simulink model "BPPID"  (R2021a)
settings: Solver=ode3  StartTime=0  StopTime=2000  FixedStep=0.05  RelTol=1e-3
settings Model: Creator=kunzhong  LastModifiedBy=sx
settings SolverCC: AlgebraicLoopSolver=TrustRegion
settings DataIOCC: SaveFormat=StructureWithTime  ReturnWorkspaceOutputs=off
settings OptimizationCC: LifeSpan=inf
settings DebuggingCC: SFExecutionAtInitializationDiag=none  SFMachineParentedDataDiag=warning  ArithmeticOperatorsInVariantConditions=warning
settings HardwareCC: ProdBitPerSizeT=32  ProdBitPerPtrDiffT=32  ProdWordSize=32  ProdHWDeviceType=Specified
settings SFSimCC: SimUseLocalCustomCode=off  CustomCodeUndefinedFunction=UseInterfaceOnly
settings RTWCC: RTWUseLocalCustomCode=off
settings CodeAppCC: StateflowObjectComments=on
settings SimscapeCC: SimscapeNormalizeSystem=off

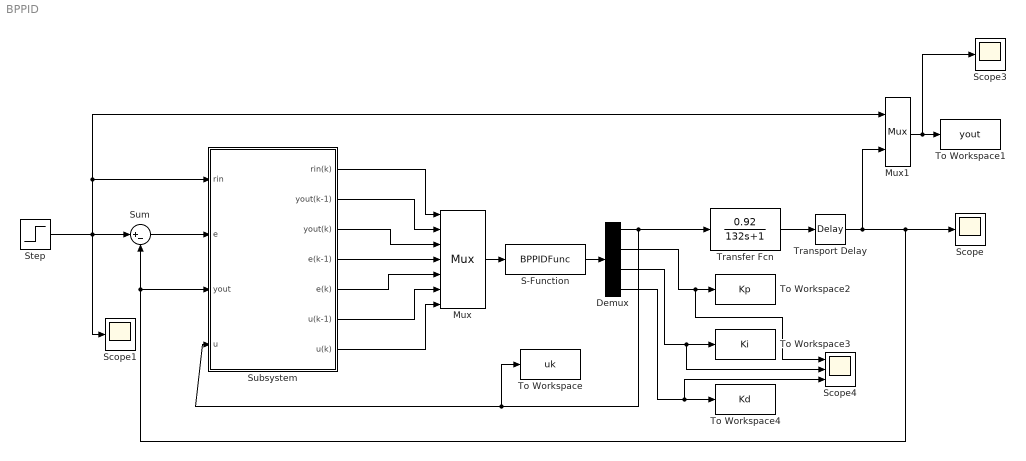
== system BPPID ==
  Demux : Demux
  Mux : Mux  Inputs=7
  Mux1 : Mux  Inputs=2
  S-Function : S-Function  FunctionName=BPPIDFunc  SFunctionDeploymentMode=off  EnableBusSupport=off
  Scope : Scope
  Scope1 : Scope
  Scope3 : Scope
  Scope4 : Scope  NumInputPorts=3
  Step : Step  SampleTime=0  ZeroCross=off
  Subsystem : Subsystem
  Sum : Sum  Inputs=|+-
  To Workspace : ToWorkspace  VariableName=uk  SaveFormat=Structure With Time  SampleTime=-1
  To Workspace1 : ToWorkspace  VariableName=yout  SaveFormat=Structure With Time  SampleTime=-1
  To Workspace2 : ToWorkspace  VariableName=Kp  SaveFormat=Structure With Time  SampleTime=-1
  To Workspace3 : ToWorkspace  VariableName=Ki  SaveFormat=Structure With Time  SampleTime=-1
  To Workspace4 : ToWorkspace  VariableName=Kd  SaveFormat=Structure With Time  SampleTime=-1
  Transfer Fcn : TransferFcn  Numerator=[0.92]  Denominator=[132 1]
  Transport Delay : TransportDelay  DelayTime=26
  wires:
  Subsystem/1(rin(k)) -> Mux/1
  Subsystem/2(yout(k-1)) -> Mux/2
  Subsystem/3(yout(k)) -> Mux/3
  Subsystem/4(e(k-1)) -> Mux/4
  Subsystem/5(e(k)) -> Mux/5
  Subsystem/6(u(k-1)) -> Mux/6
  Subsystem/7(u(k)) -> Mux/7
  Step/1 -> Scope1/1, Subsystem/1(rin), Mux1/1, Sum/1
  Sum/1 -> Subsystem/2(e)
  Mux/1 -> S-Function/1
  S-Function/1 -> Demux/1
  Demux/1 -> Subsystem/4(u), To Workspace/1, Transfer Fcn/1
  Transfer Fcn/1 -> Transport Delay/1
  Transport Delay/1 -> Mux1/2, Scope/1, Subsystem/3(yout), Sum/2
  Mux1/1 -> Scope3/1, To Workspace1/1
  Demux/2 -> Scope4/1, To Workspace2/1
  Demux/3 -> Scope4/2, To Workspace3/1
  Demux/4 -> Scope4/3, To Workspace4/1

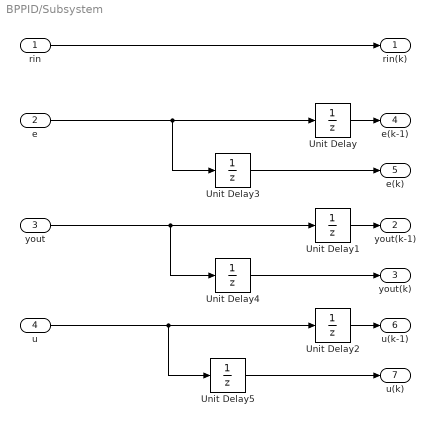
== system BPPID/Subsystem ==
  rin : Inport
  e : Inport  Port=2
  yout : Inport  Port=3
  u : Inport  Port=4
  Unit Delay{,1..5} (6 alike) : UnitDelay  SampleTime=-1  HasFrameUpgradeWarning=on
  rin(k) : Outport  VectorParamsAs1DForOutWhenUnconnected=off
  yout(k-1) : Outport  Port=2  VectorParamsAs1DForOutWhenUnconnected=off
  yout(k) : Outport  Port=3  VectorParamsAs1DForOutWhenUnconnected=off
  e(k-1) : Outport  Port=4  VectorParamsAs1DForOutWhenUnconnected=off
  e(k) : Outport  Port=5  VectorParamsAs1DForOutWhenUnconnected=off
  u(k-1) : Outport  Port=6  VectorParamsAs1DForOutWhenUnconnected=off
  u(k) : Outport  Port=7  VectorParamsAs1DForOutWhenUnconnected=off
  wires:
  rin/1 -> rin(k)/1
  Unit Delay/1 -> e(k-1)/1
  Unit Delay1/1 -> yout(k-1)/1
  Unit Delay2/1 -> u(k-1)/1
  Unit Delay3/1 -> e(k)/1
  Unit Delay4/1 -> yout(k)/1
  Unit Delay5/1 -> u(k)/1
  e/1 -> Unit Delay/1, Unit Delay3/1
  yout/1 -> Unit Delay1/1, Unit Delay4/1
  u/1 -> Unit Delay2/1, Unit Delay5/1
